simulink model "dc_motor_sim"  (R2023a)
settings: Solver=ode23tb  StartTime=0.0  StopTime=0.3  MaxStep=Ts  RelTol=1e-3
values from neighbouring files (symbols this model uses):
  gear_ratio = 31.25    [dc_motor_ini.m]
  Kd = 1.1 * Kd    [cntr_tuning_dc_motor.m]    (also in cntr_tuning_dc_motor_20D.m; dc_motor_ini.m = 1.0 * Kd)
  Kf = 60.0 / kn    (= 1.6)    [dc_motor_ini.m]
  Ki = 1.1 * Ki    [cntr_tuning_dc_motor.m]    (also in cntr_tuning_dc_motor_20D.m; dc_motor_ini.m = 1.0 * Ki)
  Kp = 1.2 * Kp    [cntr_tuning_dc_motor.m]    (also in cntr_tuning_dc_motor_20D.m; dc_motor_ini.m = 1.0 * Kp; modelling_and_cntrl_tuning_dc_motor_25D.m = 8)
  Ts = 5e-4    (= 0.0005)    [cntr_tuning_dc_motor.m]    (also in cntr_tuning_dc_motor_20D.m; dc_motor_ini.m = 0.001; design_upsampling_filter.m = 0.0002; modelling_and_cntrl_tuning_dc_motor_25D.m = mean(diff(data.time)))
libraries: cstblocks x8
settings Model: Creator=Michael Peter  LastModifiedBy=Michael Peter

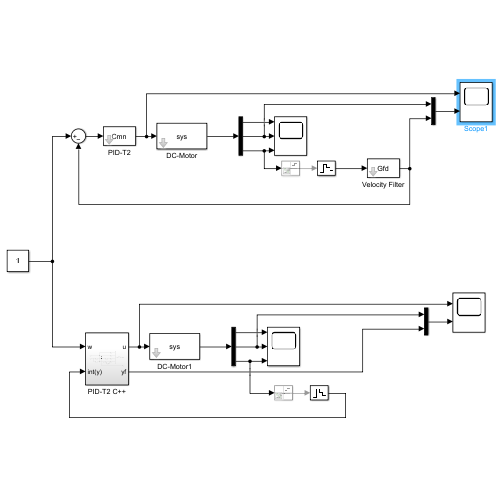
[thumbnail: Simulink's stored preview of the top-level diagram]
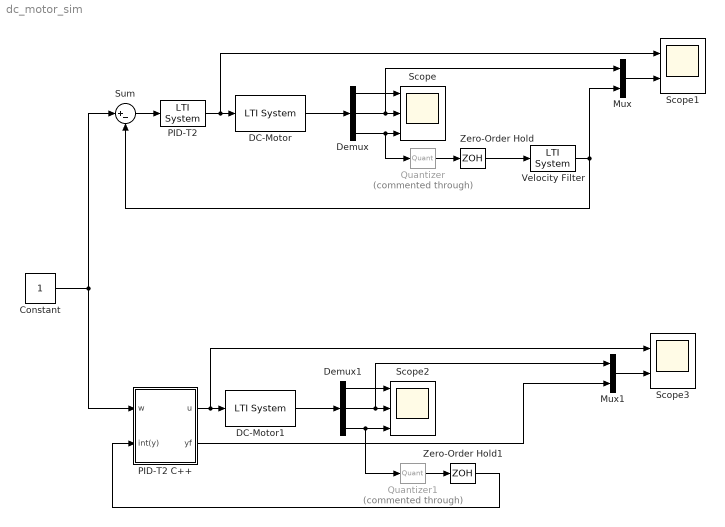
== system dc_motor_sim ==
  Constant : Constant
  DC-Motor : cstblocks/LTI System  sys=sys  IC=[]
  DC-Motor1 : cstblocks/LTI System  sys=sys  IC=[]
  Demux : Demux  Outputs=3
  Demux1 : Demux  Outputs=3
  Mux : Mux  Inputs=2
  Mux1 : Mux  Inputs=2
  PID-T2 : cstblocks/LTI System  sys=Cmn  IC=[]
  PID-T2 C++ : Subsystem
  Quantizer : Quantizer  Commented=through  QuantizationInterval=1 / (gear_ratio*20)
  Quantizer1 : Quantizer  Commented=through  QuantizationInterval=1 / (gear_ratio*20)
  Scope : Scope  NumInputPorts=3
  Scope1 : Scope  NumInputPorts=2
  Scope2 : Scope  NumInputPorts=3
  Scope3 : Scope  NumInputPorts=2
  Sum : Sum  Inputs=|+-
  Velocity Filter : cstblocks/LTI System  sys=Gfd  IC=[]
  Zero-Order Hold : ZeroOrderHold  SampleTime=Ts
  Zero-Order Hold1 : ZeroOrderHold  SampleTime=Ts
  wires:
  DC-Motor/1 -> Demux/1
  Demux/3 -> Quantizer/1, Scope/3
  Zero-Order Hold/1 -> Velocity Filter/1
  PID-T2/1 -> Scope1/1, DC-Motor/1
  Velocity Filter/1 -> Mux/2, Sum/2
  Sum/1 -> PID-T2/1
  Demux/1 -> Scope/1
  Demux/2 -> Mux/1, Scope/2
  Mux/1 -> Scope1/2
  Quantizer/1 -> Zero-Order Hold/1
  Mux1/1 -> Scope3/2
  Demux1/2 -> Scope2/2, Mux1/1
  Demux1/1 -> Scope2/1
  Constant/1 -> PID-T2 C++/1(w), Sum/1
  PID-T2 C++/2(yf) -> Mux1/2
  Demux1/3 -> Quantizer1/1, Scope2/3
  DC-Motor1/1 -> Demux1/1
  PID-T2 C++/1(u) -> Scope3/1, DC-Motor1/1
  Quantizer1/1 -> Zero-Order Hold1/1
  Zero-Order Hold1/1 -> PID-T2 C++/2(int(y))

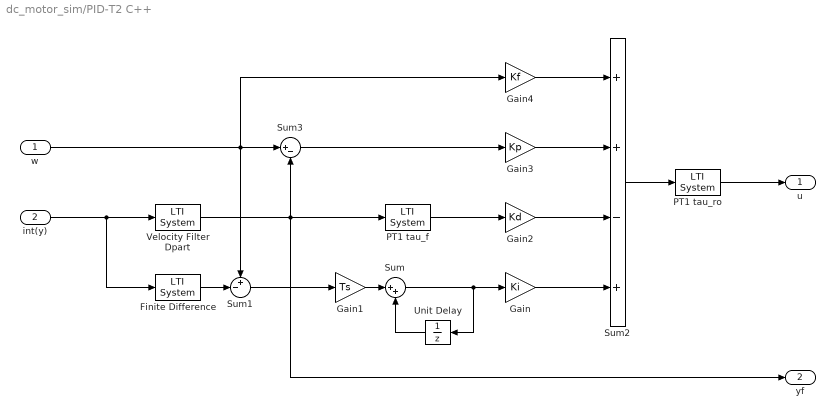
== system dc_motor_sim/PID-T2 C++ ==
  w : Inport
  int(y) : Inport  Port=2
  Finite Difference : cstblocks/LTI System  sys=Gd  IC=[]
  Gain : Gain  Gain=Ki
  Gain1 : Gain  Gain=Ts
  Gain2 : Gain  Gain=Kd
  Gain3 : Gain  Gain=Kp
  Gain4 : Gain  Gain=Kf
  PT1 tau_f : cstblocks/LTI System  sys=G_tau_f  IC=[]
  PT1 tau_ro : cstblocks/LTI System  sys=G_tau_ro  IC=[]
  Sum : Sum  Inputs=|++
  Sum1 : Sum  Inputs=+-|
  Sum2 : Sum  Inputs=++-+
  Sum3 : Sum  Inputs=|+-
  Unit Delay : UnitDelay  SampleTime=Ts  HasFrameUpgradeWarning=on
  Velocity Filter Dpart : cstblocks/LTI System  sys=Gfd  IC=[]
  u : Outport
  yf : Outport  Port=2
  wires:
  PT1 tau_ro/1 -> u/1
  Sum2/1 -> PT1 tau_ro/1
  Gain4/1 -> Sum2/1
  Gain3/1 -> Sum2/2
  Gain2/1 -> Sum2/3
  Gain/1 -> Sum2/4
  Sum3/1 -> Gain3/1
  PT1 tau_f/1 -> Gain2/1
  Velocity Filter Dpart/1 -> PT1 tau_f/1, Sum3/2, yf/1
  w/1 -> Sum1/1, Sum3/1, Gain4/1
  Sum/1 -> Unit Delay/1, Gain/1
  Unit Delay/1 -> Sum/2
  Gain1/1 -> Sum/1
  Finite Difference/1 -> Sum1/2
  int(y)/1 -> Velocity Filter Dpart/1, Finite Difference/1
  Sum1/1 -> Gain1/1
